simulink model "model1"  (Simulink 6.6)
settings: Solver=ode45  StartTime=0.0  StopTime=12  RelTol=1e-3
settings Model: Creator=mxkana  LastModifiedBy=mxkana

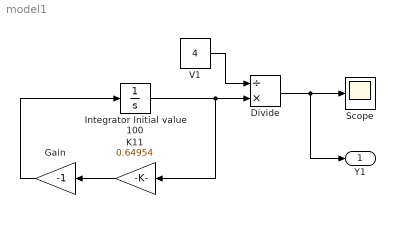
== system model1 ==
  Divide : Product  Inputs=/*  OutScaling=2^-10
  Gain : Gain  Orientation=left  Gain=-1
  Integrator Initial value 100 : Integrator  InitialCondition=100
  K11 : Gain  Orientation=left  Gain=0.64954
  Scope : Scope
  V1 : Constant  Value=4
  Y1 : Outport
  wires:
  Integrator Initial value 100/1 -> K11/1, Divide/2
  K11/1 -> Gain/1
  Gain/1 -> Integrator Initial value 100/1
  V1/1 -> Divide/1
  Divide/1 -> Scope/1, Y1/1
